simulink model "logistic_map"  (R2024b)
settings: Solver=VariableStepAuto  StartTime=0.0  StopTime=10.0  RelTol=1e-3
settings Model: Creator=Botló  LastModifiedBy=Botló

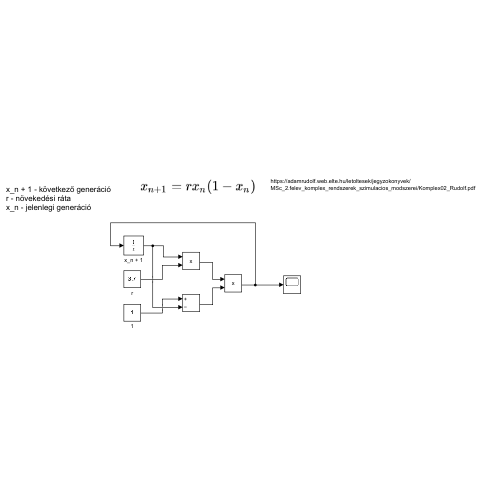
[thumbnail: Simulink's stored preview of the top-level diagram]
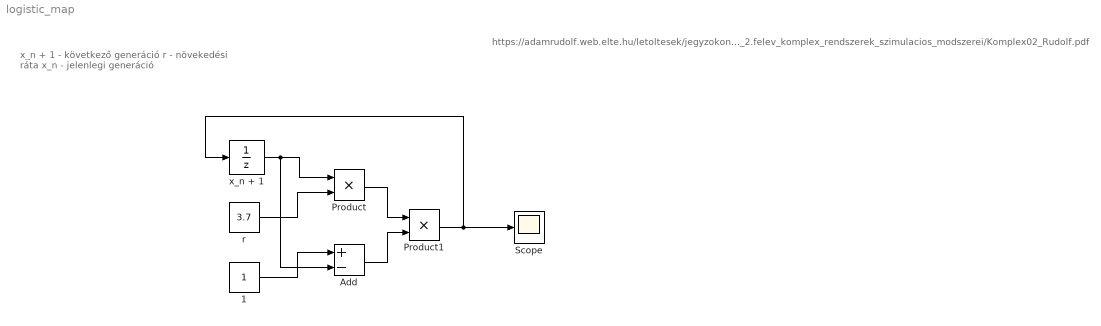
== system logistic_map ==
  note: x_n + 1 - következő generáció
      | r - növekedési ráta
      | x_n - jelenlegi generáció
  note: https://adamrudolf.web.elte.hu/letoltesek/jegyzokonyvek/MSc_2.felev_komplex_rendszerek_szimulacios_modszerei/Komplex02_Rudolf.pdf
  1 : Constant
  Add : Sum  Inputs=+-
  Product : Product
  Product1 : Product
  Scope : Scope
  r : Constant  Value=3.7
  x_n + 1 : UnitDelay  InitialCondition=0.5  SampleTime=-1  HasFrameUpgradeWarning=on
  wires:
  x_n + 1/1 -> Add/2, Product/1
  r/1 -> Product/2
  Product/1 -> Product1/1
  1/1 -> Add/1
  Add/1 -> Product1/2
  Product1/1 -> Scope/1, x_n + 1/1
